simulink model "simulink_pratica6"  (R2021b)
settings: Solver=VariableStepAuto  StartTime=0.0  StopTime=24  RelTol=1e-3
settings Model: Creator=13676840  LastModifiedBy=13676840

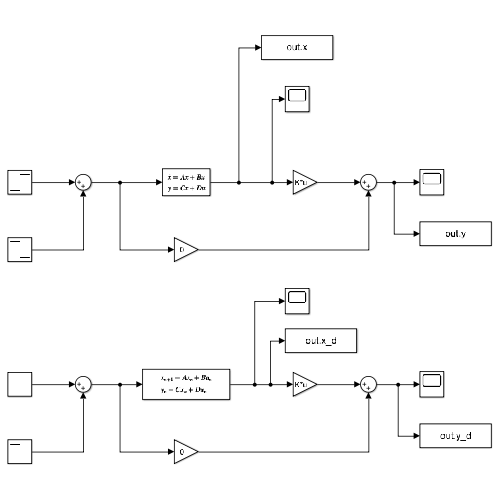
[thumbnail: Simulink's stored preview of the top-level diagram]
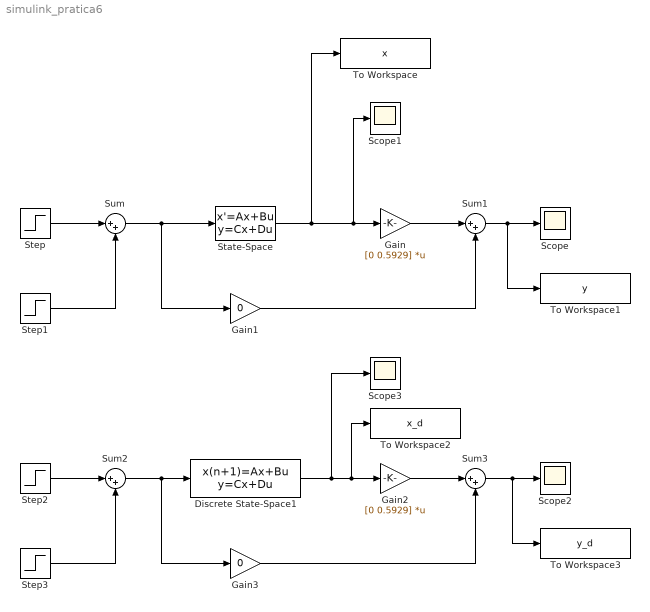
== system simulink_pratica6 ==
  Discrete State-Space1 : DiscreteStateSpace  A=[0.8672 -0.0496; 0.0836 0.9977]  B=[0.0836; 0.0038]  C=[1 0; 0 1]  D=[0;0]  SampleTime=0.0897
  Gain : Gain  Gain=[0 0.5929]  Multiplication=Matrix(K*u)
  Gain1 : Gain  Gain=0
  Gain2 : Gain  Gain=[0 0.5929]  Multiplication=Matrix(K*u)
  Gain3 : Gain  Gain=0
  Scope{,1..3} (4 alike) : Scope
  State-Space : StateSpace  A=[-1.56 -0.5929; 1 0]  B=[1; 0]  C=[1 0; 0 1]  D=[0;0]  InitialCondition=0
  Step : Step  Time=0  After=1.17  SampleTime=0
  Step1 : Step  Time=12  After=-0.15  SampleTime=0
  Step2 : Step  Time=0  After=1.17  SampleTime=0
  Step3 : Step  Time=12  After=-0.15  SampleTime=0
  Sum{,1..3} (4 alike) : Sum  Inputs=|++
  To Workspace : ToWorkspace  VariableName=x  SaveFormat=Timeseries  SampleTime=-1
  To Workspace1 : ToWorkspace  VariableName=y  SaveFormat=Timeseries  SampleTime=-1
  To Workspace2 : ToWorkspace  VariableName=x_d  SaveFormat=Timeseries  SampleTime=-1
  To Workspace3 : ToWorkspace  VariableName=y_d  SaveFormat=Timeseries  SampleTime=-1
  wires:
  Step/1 -> Sum/1
  Sum/1 -> State-Space/1, Gain1/1
  Step1/1 -> Sum/2
  State-Space/1 -> To Workspace/1, Scope1/1, Gain/1
  Gain/1 -> Sum1/1
  Gain1/1 -> Sum1/2
  Sum1/1 -> To Workspace1/1, Scope/1
  Gain3/1 -> Sum3/2
  Gain2/1 -> Sum3/1
  Discrete State-Space1/1 -> To Workspace2/1, Gain2/1, Scope3/1
  Step3/1 -> Sum2/2
  Step2/1 -> Sum2/1
  Sum3/1 -> To Workspace3/1, Scope2/1
  Sum2/1 -> Gain3/1, Discrete State-Space1/1
